simulink model "mergedemo"  (R2019b)
settings: Solver=VariableStepDiscrete  StartTime=0.0  StopTime=20  MaxStep=.1  RelTol=1e-3  AbsTol=1e-6
libraries: simulink x1
Description:
  | Merging Signals
  | 
  | This model shows the following Simulink(R) concepts:
  | 
  |  * Conditionally executed subsystems
  |  * Logical Operator block
  |  * Boolean signals in Simulink
  |  * Creating alternately enabling subsystems using the Merge block
settings Model: ExtModeTrigMode=oneshot  ExtModeArmWhenConnect=off  ExtModeAutoUpdateStatusClock=off  Creator=The MathWorks, Inc.  LastModifiedBy=bhisma
settings SolverCC: AutoScaleAbsTol=off
settings DataIOCC: SaveFormat=Array
settings OptimizationCC: BlockReduction=off  ExpressionDepthLimit=2147483647  InitFltsAndDblsToZero=on  LifeSpan=inf  BufferReusableBoundary=off
settings DebuggingCC: SaveWithParameterizedLinksMsg=none  SignalResolutionControl=TryResolveAllWithWarning  MultiTaskDSMMsg=warning  MultiTaskCondExecSysMsg=none  IntegerOverflowMsg=none  FcnCallInpInsideContextMsg=warning  BusObjectLabelMismatch=none  AllowSymbolicDim=off  StateNameClashWarn=warning  SFUnexpectedBacktrackingDiag=warning  SFNoUnconditionalDefaultTransitionDiag=warning  SFExecutionAtInitializationDiag=none  IntegerSaturationMsg=none  ArithmeticOperatorsInVariantConditions=warning
settings HardwareCC: ProdBitPerPointer=32  ProdBitPerSizeT=32  ProdBitPerPtrDiffT=32  ProdLargestAtomicFloat=None  ProdIntDivRoundTo=Undefined  ProdEndianess=Unspecified  ProdWordSize=32  ProdHWDeviceType=32-bit Generic  TargetUnknown=on
settings ModelReferenceCC: PropagateSignalLabelsOutOfModel=off
settings SFSimCC: SimUseLocalCustomCode=off  CustomCodeUndefinedFunction=UseInterfaceOnly
settings RTWCC: Description=Generic Real-Time Target  RTWUseLocalCustomCode=off
settings CodeAppCC: StateflowObjectComments=on
settings GRTTargetCC: TargetFcnLib=ansi_tfl_tmw.mat  TargetLangStandard=C89/C90 (ANSI)  GeneratePreprocessorConditionals=Disable all  CombineOutputUpdateFcns=off  GRTInterface=on
settings ConfigComp: CovMetricSettings=dw  CovHtmlReporting=on  CovSaveCumulativeToWorkspaceVar=on  CovSaveSingleToWorkspaceVar=on  CovExternalEMLEnable=off

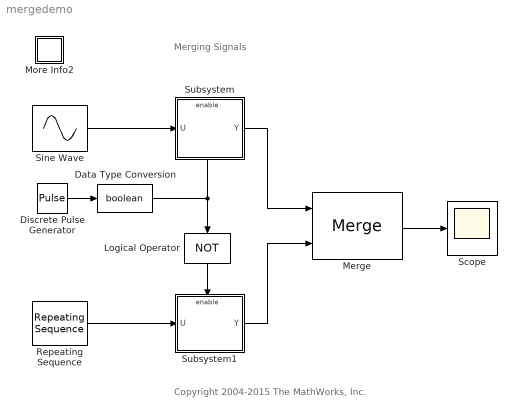
== system mergedemo ==
  note: Merging Signals
  note: Copyright 2004-2015 The MathWorks, Inc.
  Data Type Conversion : DataTypeConversion  OutDataTypeStr=boolean  SaturateOnIntegerOverflow=on  RndMeth=Zero
  Discrete Pulse Generator : DiscretePulseGenerator  SampleTime=5
  Logical Operator : Logic  Operator=NOT  Inputs=1  OutDataTypeStr=boolean
  Merge : Merge
  More Info2 : Subsystem
      settings: OpenFcn=showdemo(bdroot(gcs))
      mask Display: disp('?')
  Repeating Sequence : simulink/Sources/Repeating Sequence  rep_seq_t=[0 1]  rep_seq_y=[0 2]
  Scope : Scope
  Sine Wave : Sin  Frequency=pi  SampleTime=0
  Subsystem : Subsystem  Tag=MergeExample  TreatAsAtomicUnit=on
  Subsystem1 : Subsystem  Tag=MergeExample  TreatAsAtomicUnit=on
  wires:
  Sine Wave/1 -> Subsystem/1(U)
  Subsystem/1(Y) -> Merge/1
  Subsystem1/1(Y) -> Merge/2
  Logical Operator/1 -> Subsystem1/Enable
  Discrete Pulse Generator/1 -> Data Type Conversion/1
  Repeating Sequence/1 -> Subsystem1/1(U)
  Merge/1 -> Scope/1
  Data Type Conversion/1 -> Logical Operator/1, Subsystem/Enable

== system mergedemo/More Info2 ==

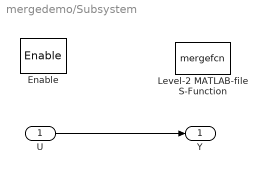
== system mergedemo/Subsystem ==
  U : Inport
  Enable : EnablePort  StatesWhenEnabling=reset
  Level-2 MATLAB-file S-Function : M-S-Function  FunctionName=mergefcn
  Y : Outport  VectorParamsAs1DForOutWhenUnconnected=off
  wires:
  U/1 -> Y/1

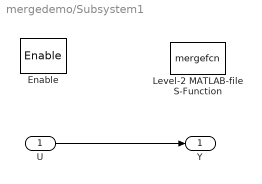
== system mergedemo/Subsystem1 ==
  U : Inport
  Enable : EnablePort  StatesWhenEnabling=reset
  Level-2 MATLAB-file S-Function : M-S-Function  FunctionName=mergefcn
  Y : Outport  VectorParamsAs1DForOutWhenUnconnected=off
  wires:
  U/1 -> Y/1
